simulink model "pitcher"  (R2020a)
settings: Solver=VariableStepAuto  StartTime=0.0  StopTime=10.0  RelTol=1e-3
undefined symbols (not defined in the file or in its folder): A2, B2, C2, D2, Earth, WGS84
libraries: aerolibfltsims x2, aerolibtransform2 x1, simulink x1
settings Model: Creator=Khojasteh Mirza  LastModifiedBy=Khojasteh Mirza

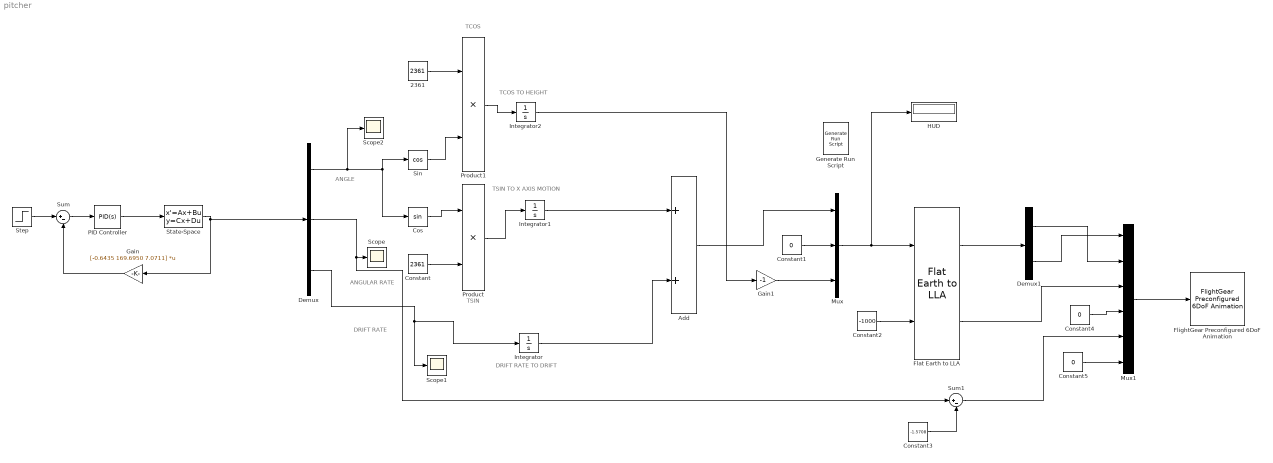
== system pitcher ==
  note: DRIFT RATE TO DRIFT
  note: TSIN TO X AXIS MOTION
  note: TCOS
  note: TSIN
  note: ANGULAR RATE
  note: DRIFT RATE
  note: ANGLE
  note: TCOS TO HEIGHT
  2361 : Constant  Value=2361
  Add : Sum
  Constant : Constant  Value=2361
  Constant1 : Constant  Value=0
  Constant2 : Constant  Value=-1000
  Constant3 : Constant  Value=-1.5708
  Constant4 : Constant  Value=0
  Constant5 : Constant  Value=0
  Cos : Trigonometry
  Demux : Demux  Outputs=3
  Demux1 : Demux  Outputs=2
  Flat Earth to LLA : aerolibtransform2/Flat Earth to LLA  units=Metric (MKS)  ptype=Earth (WGS84)  F=1/298.257223563  R=6378137  refPosPort=off  LL0=[0 10]  psi=0
  FlightGear Preconfigured 6DoF Animation : aerolibfltsims/FlightGear Preconfigured 6DoF Animation  xFlightGearVersion=v3.2  DestinationIpAddress=127.0.0.1  DestinationPort=5502  SampleTime=1/30  packetVersion=24
  Gain : Gain  Gain=[-0.6435 169.6950 7.0711]  Multiplication=Matrix(K*u)
  Gain1 : Gain  Gain=-1
  Generate Run Script : aerolibfltsims/Generate Run Script  Architecture=Default  dataFlow=Send  GeometryModelName=HL20  AirportId=KSFO  RunwayId=10L  InitialAltitude=7224  InitialHeading=113  OffsetDistance=4.72  OffsetAzimuth=0  InstallScenery=off  DisableShaders=off  OriginAddress=127.0.0.1  DestinationPort=5502  OriginPort=5505  LocalAddress=127.0.0.1  OutputFileName=runfgpitch.bat  FlightGearBaseDirectory=C:\Program Files\FlightGear 2020.3.2
  HUD : Display
  Integrator : Integrator
  Integrator1 : Integrator
  Integrator2 : Integrator
  Mux : Mux  Inputs=3
  Mux1 : Mux  Inputs=6
  PID Controller : simulink/Continuous/PID Controller  Controller=PID  Form=Parallel  TimeDomain=Continuous-time  UseExternalTs=off  SampleTime=-1  IntegratorMethod=Forward Euler  FilterMethod=Forward Euler  ControllerParametersSource=internal  P=0.496212436803171  I=0.33424014776781  D=0.131574819555698  UseFilter=on  N=4.3699731980731  TunerSelectOption=Transfer Function Based (PID Tuner App)  InitialConditionSource=internal  InitialConditionForIntegrator=0  InitialConditionForFilter=0  DifferentiatorICPrevScaledInput=0  ExternalReset=none  TrackingMode=off  Kt=1  LimitOutput=on  UpperSaturationLimit=0.43  LowerSaturationLimit=-0.43  LinearizeAsGain=on  AntiWindupMode=none  Kb=1  POutMin=[]  POutMax=[]  IOutMin=[]  IOutMax=[]  DOutMin=[]  DOutMax=[]  NOutMin=[]  NOutMax=[]  SumOutMin=[]  SumOutMax=[]  SaturationOutMin=[]  SaturationOutMax=[]  PParamMin=[]  PParamMax=[]  IParamMin=[]  IParamMax=[]  DParamMin=[]  DParamMax=[]  NParamMin=[]  NParamMax=[]  KbParamMin=[]  KbParamMax=[]  KtParamMin=[]  KtParamMax=[]  KbOutMin=[]  KbOutMax=[]  KtOutMin=[]  KtOutMax=[]  IntegratorOutMin=[]  IntegratorOutMax=[]  FilterOutMin=[]  FilterOutMax=[]  SumI1OutMin=[]  SumI1OutMax=[]  SumI2OutMin=[]  SumI2OutMax=[]  SumI3OutMin=[]  SumI3OutMax=[]  SumI4OutMin=[]  SumI4OutMax=[]  SumDOutMin=[]  SumDOutMax=[]  DifferentiatorOutMin=[]  DifferentiatorOutMax=[]  FilterDiffOutCoefMin=[]  FilterDiffOutCoefMax=[]  ReciprocalOutMin=[]  ReciprocalOutMax=[]  SumDenOutMin=[]  SumDenOutMax=[]  SumNumOutMin=[]  SumNumOutMax=[]  DivideOutMin=[]  DivideOutMax=[]  UdiffTsProdOutMin=[]  UdiffTsProdOutMax=[]  NTsProdOutMin=[]  NTsProdOutMax=[]  UintegralTsProdOutMin=[]  UintegralTsProdOutMax=[]  UngainTsProdOutMin=[]  UngainTsProdOutMax=[]  IntegratorContinuousStateAttributes=''  IntegratorStateMustResolveToSignalObject=off  IntegratorRTWStateStorageClass=Auto  FilterContinuousStateAttributes=''  FilterStateMustResolveToSignalObject=off  FilterRTWStateStorageClass=Auto  ParallelPVariant=InternalParameters  IdealPVariant=Disabled  IVariant=InternalParameters  DVariant=InternalParameters  IntegratorVariant=Continuous  SatVariant=Enabled  AWVariant=Passthrough  PCopyVariant=Disabled  TRVariant=Disabled  FdbkBlocksVariant=Forward  IdealPFdbkVariant=Disabled  SatFdbkVariant=Disabled  DerivativeFilterVariant=ContFilter  NVariant=InternalParameters  NCopyVariant=Disabled  FilterICVariant=InternalICsFilter  IntegratorICVariant=InternalICs  ExternalResetVariant=Disabled  TRSumVariant=Passthrough  SumFdbkVariant=Disabled  SumVariant=Sum_PID  TsampFilterVariant=InternalTs  TsampNgainVariant=Passthrough  TsampIntegralVariant=Passthrough
  Product : Product
  Product1 : Product
  Scope : Scope
  Scope1 : Scope
  Scope2 : Scope
  Sin : Trigonometry  Operator=cos
  State-Space : StateSpace  A=A2  B=B2  C=C2  D=D2  InitialCondition=0  ContinuousStateAttributes={'AoA','Pitch_Rate','Pitch_Angle'}
  Step : Step  SampleTime=0
  Sum : Sum  Inputs=|+-
  Sum1 : Sum  Inputs=|+-
  wires:
  State-Space/1 -> Gain/1, Demux/1
  Step/1 -> Sum/1
  Gain/1 -> Sum/2
  Sum/1 -> PID Controller/1
  PID Controller/1 -> State-Space/1
  Integrator2/1 -> Gain1/1
  Sum1/1 -> Mux1/5
  Flat Earth to LLA/2 -> Mux1/3
  Mux1/1 -> FlightGear Preconfigured 6DoF Animation/1
  Flat Earth to LLA/1 -> Demux1/1
  Demux1/2 -> Mux1/1
  Constant3/1 -> Sum1/2
  Constant4/1 -> Mux1/4
  Constant5/1 -> Mux1/6
  Mux/1 -> HUD/1, Flat Earth to LLA/1
  Integrator/1 -> Add/2
  Add/1 -> Mux/1
  Demux/3 -> Scope1/1, Integrator/1
  Constant2/1 -> Flat Earth to LLA/2
  Product1/1 -> Integrator2/1
  Demux1/1 -> Mux1/2
  Product/1 -> Integrator1/1
  Gain1/1 -> Mux/3
  Constant/1 -> Product/2
  Demux/1 -> Scope2/1, Cos/1, Sin/1
  Sin/1 -> Product1/2
  2361/1 -> Product1/1
  Cos/1 -> Product/1
  Integrator1/1 -> Add/1
  Constant1/1 -> Mux/2
  Demux/2 -> Sum1/1, Scope/1
